simulink model "Test_Character_Table"  (Simulink 8.1)
settings: Solver=ode45  SolverMode=SingleTasking  StartTime=0.0  StopTime=2  RelTol=1e-3
undefined symbols (not defined in the file): HEIGHT, hot, PERCENT, POS_X, POS_Y, vect, WIDTH
libraries: dspsnks4 x2, Computer_Library x1
settings Model: Creator=N  LastModifiedBy=uzivatel
settings OptimizationCC: BlockReduction=off  BooleanDataType=off  ExpressionDepthLimit=128
settings DebuggingCC: SaveWithParameterizedLinksMsg=none  SignalResolutionControl=TryResolveAllWithWarning  SolverPrmCheckMsg=none  MultiTaskDSMMsg=warning  MultiTaskCondExecSysMsg=none  FcnCallInpInsideContextMsg=EnableAllAsError  StrictBusMsg=None
settings HardwareCC: TargetUnknown=on
settings RTWCC: IncludeERTFirstTime=on
settings GRTTargetCC: CombineOutputUpdateFcns=on  GRTInterface=off

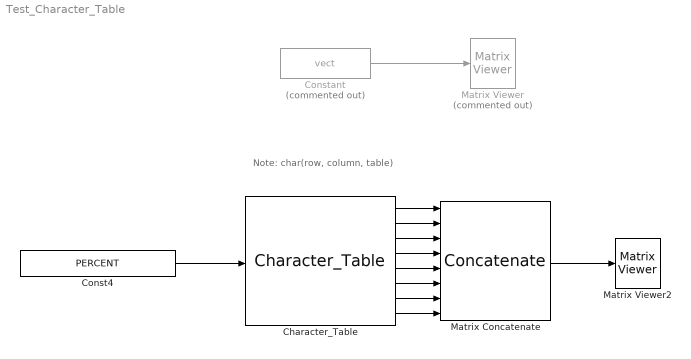
== system Test_Character_Table ==
  note: Note: char(row, column, table)
  Character_Table : Computer_Library/Character_Table
  Const4 : Constant  Value=PERCENT  OutDataTypeStr=uint8
  Constant : Constant  Commented=on  Value=vect  OutDataTypeStr=uint8
  Matrix Concatenate : Concatenate  NumInputs=8  Mode=Multidimensional array  ConcatenateDimension=2
  Matrix Viewer : dspsnks4/Matrix Viewer  Commented=on  ImageParams=off  CMapStr=hot(256)  AxisColorbar=on  AxisParams=off  AxisOrigin=Upper left corner  XLabel=X-axis  YLabel=Y-axis  ZLabel=Z-axis  FigPos=[500 1000 1100 15]  AxisZoom=on
      settings: YMin=0  YMax=1.0
  Matrix Viewer2 : dspsnks4/Matrix Viewer  ImageParams=off  CMapStr=hot(256)  AxisColorbar=on  AxisParams=off  AxisOrigin=Upper left corner  XLabel=X-axis  YLabel=Y-axis  ZLabel=Z-axis  FigPos=[POS_X POS_Y WIDTH HEIGHT]  AxisZoom=on
      settings: YMin=0  YMax=1.0
  wires:
  Constant/1 -> Matrix Viewer/1
  Matrix Concatenate/1 -> Matrix Viewer2/1
  Character_Table/1 -> Matrix Concatenate/1
  Character_Table/2 -> Matrix Concatenate/2
  Character_Table/3 -> Matrix Concatenate/3
  Character_Table/4 -> Matrix Concatenate/4
  Character_Table/5 -> Matrix Concatenate/5
  Character_Table/6 -> Matrix Concatenate/6
  Character_Table/7 -> Matrix Concatenate/7
  Character_Table/8 -> Matrix Concatenate/8
  Const4/1 -> Character_Table/1
